simulink model "dynamic_system_alone"  (R2024b)
settings: Solver=VariableStepAuto  StartTime=0.0  StopTime=10.0  RelTol=1e-3
libraries: robotmaniplib x4
settings Model: Creator=spenu  LastModifiedBy=spenu

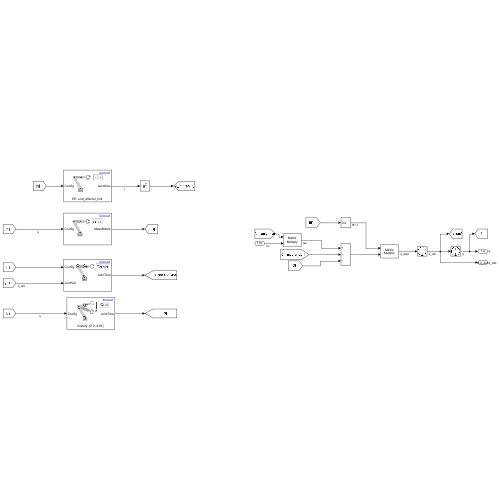
[thumbnail: Simulink's stored preview of the top-level diagram]
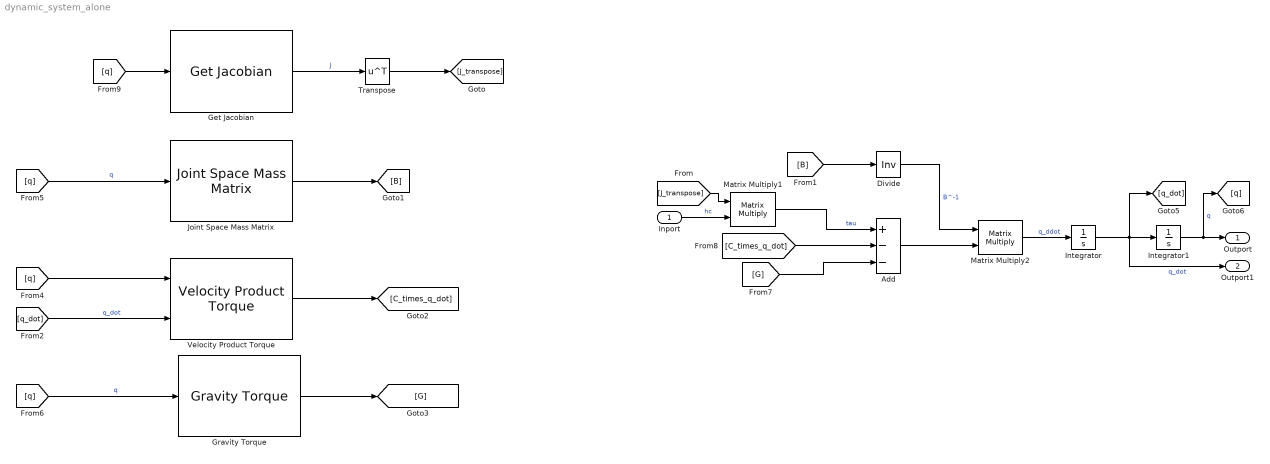
== system dynamic_system_alone ==
  Inport : Inport  PortDimensions=[6,1]
  Add : Sum  Inputs=+--
  Divide : Product  Inputs=/  Multiplication=Matrix(*)
  Get Jacobian : robotmaniplib/Get Jacobian  RigidBodyTree=kinova1  EndEffector=end_effector_link  SimulateUsing=Interpreted execution
  Gravity Torque : robotmaniplib/Gravity Torque  RigidBodyTree=kinova1  SimulateUsing=Interpreted execution
  Integrator : Integrator  WrapState=on  WrappedStateUpperValue=2*pi  WrappedStateLowerValue=-2*pi
  Integrator1 : Integrator  WrapState=on
  Joint Space Mass Matrix : robotmaniplib/Joint Space Mass Matrix  RigidBodyTree=kinova1  SimulateUsing=Interpreted execution
  Matrix Multiply1 : Product  Multiplication=Matrix(*)
  Matrix Multiply2 : Product  Multiplication=Matrix(*)
  Transpose : Math  Operator=transpose
  Velocity Product Torque : robotmaniplib/Velocity Product Torque  RigidBodyTree=kinova1  SimulateUsing=Interpreted execution
  Outport : Outport  SignalName=q  PortDimensions=[6,1]
  Outport1 : Outport  Port=2  SignalName=q_dot  PortDimensions=[6,1]
  wires:
  [C_times_q_dot] -> Add/2
  [G] -> Add/3
  [B] -> Divide/1
  Divide/1 -> Matrix Multiply2/1  "B^-1"
  Add/1 -> Matrix Multiply2/2
  Get Jacobian/1 -> Transpose/1  "J"
  [q] -> Get Jacobian/1
  Transpose/1 -> [J_transpose]
  [q] -> Joint Space Mass Matrix/1  "q"
  [q_dot] -> Velocity Product Torque/2  "q_dot"
  Gravity Torque/1 -> [G]
  Velocity Product Torque/1 -> [C_times_q_dot]
  Joint Space Mass Matrix/1 -> [B]
  [q] -> Velocity Product Torque/1
  [q] -> Gravity Torque/1  "q"
  Matrix Multiply2/1 -> Integrator/1  "q_ddot"
  Integrator/1 -> Outport1/1, [q_dot], Integrator1/1  "q_dot"
  Integrator1/1 -> [q], Outport/1  "q"
  Inport/1 -> Matrix Multiply1/2  "hc"
  [J_transpose] -> Matrix Multiply1/1
  Matrix Multiply1/1 -> Add/1  "tau"
